simulink model "CHB2simulation2"  (R2014a)
settings: Solver=ode1  StartTime=0.0  StopTime=Tsim  FixedStep=Ts  RelTol=1e-3
InitFcn:
  | GlobalParam2;
values from neighbouring files (symbols this model uses):
  Cdc = 680e-6    (= 0.00068)    [GlobalParam2.m]
  Ideal = 1    [GlobalParam2.m]
  Rdc = 910e3    (= 910000)    [GlobalParam2.m]
  tetaa = 0    [GlobalParam2.m]
  tetab = 240    [GlobalParam2.m]
  tetac = 120    [GlobalParam2.m]
  Ts = Tm/100    (= 0.0002)    [GlobalParam2.m]
  Vdc = Vs    [GlobalParam2.m]
  Vs = 220*sqrt(2)    [GlobalParam2.m]
  we = 2*pi*fe    (= 314.159265359)    [GlobalParam2.m]
undefined symbols (not defined in the file or in its folder): Lf
libraries: powerlib x34
settings Model: Creator=Leocompa  LastModifiedBy=Leocompa

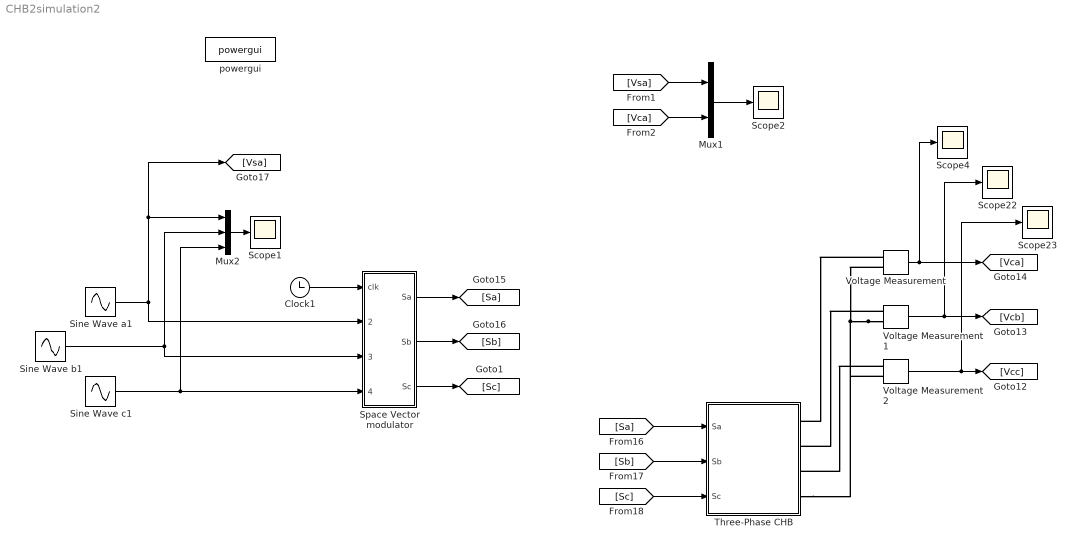
== system CHB2simulation2 ==
  Clock1 : Clock
  Mux1 : Mux  Inputs=2
  Mux2 : Mux  Inputs=3
  Scope{1..2,4,22..23} (5 alike) : Scope
      Scope1 settings: YMin=-2500  YMax=37500  SaveName=vca1
      Scope2 settings: YMin=-350  YMax=350  SaveName=vca2
      Scope22 settings: YMin=-2500  YMax=37500  SaveName=vcb
      Scope23 settings: YMin=-2500  YMax=37500  SaveName=vcc
      Scope4 settings: YMin=-2500  YMax=37500  SaveName=vca
  Sine Wave a1 : Sin  Amplitude=Vs  Frequency=we  Phase=tetaa  SampleTime=0
  Sine Wave b1 : Sin  Amplitude=Vs  Frequency=we  Phase=tetab*pi/180  SampleTime=0
  Sine Wave c1 : Sin  Amplitude=Vs  Frequency=we  Phase=tetac*pi/180  SampleTime=0
  Space Vector modulator : Subsystem
  Three-Phase CHB : Subsystem
  Voltage Measurement : powerlib/Measurements/Voltage Measurement  PhasorSimulation=off  OutputType=Complex  PSBequivalent=0
  Voltage Measurement1 : powerlib/Measurements/Voltage Measurement  PhasorSimulation=off  OutputType=Complex  PSBequivalent=0
  Voltage Measurement2 : powerlib/Measurements/Voltage Measurement  PhasorSimulation=off  OutputType=Complex  PSBequivalent=0
  powergui : powerlib/powergui  SimulationMode=Discrete  SolverType=Backward Euler  SampleTime=Ts  frequency=60  SPID=off  DisableSnubberDevices=off  DisableRonSwitches=off  DisableVfSwitches=off  SwTol=0  Interpol=off  DisplayEquations=off  Ts=0  methode=off  frequencyindice=0  Pbase=100e6  ErrMax=1e-4  Iterations=50  UnitsV=kV  UnitsW=MW  FunctionMessages=off  echomessages=off  HookPort=off  EnableUseOfTLC=off  x0status=blocks  RestoreLinks=warning  ResistiveCurrentMeasurement=off  Frange=[0:2:500]  Ylog=off  Xlog=on  ShowGrid=off  save=off  variable=ZData  structure=sa11  ZoomFFT=off  StartTime=0  cycles=8  DisplayStyle=1  fundamental=50  FreqAxis=off  MaxFrequency=10000  frequencyindicesteady=1  RmsSteady=1  display=off
  wires:
  Voltage Measurement/1 -> [Vca], Scope4/1
  Voltage Measurement2/1 -> Scope23/1, [Vcc]
  [Sa] -> Three-Phase CHB/1(Sa)
  [Sb] -> Three-Phase CHB/2(Sb)
  [Sc] -> Three-Phase CHB/3(Sc)
  Voltage Measurement1/1 -> [Vcb], Scope22/1
  [Vsa] -> Mux1/1
  [Vca] -> Mux1/2
  Mux1/1 -> Scope2/1
  Sine Wave a1/1 -> Space Vector modulator/2(vca ref), [Vsa], Mux2/1
  Sine Wave b1/1 -> Mux2/2, Space Vector modulator/3(vcb ref1)
  Sine Wave c1/1 -> Mux2/3, Space Vector modulator/4(vcc ref2)
  Mux2/1 -> Scope1/1
  Clock1/1 -> Space Vector modulator/1(clk)
  Space Vector modulator/3(Sc) -> [Sc]
  Space Vector modulator/2(Sb) -> [Sb]
  Space Vector modulator/1(Sa) -> [Sa]
  connections:
  Voltage Measurement1/LConn2 -- Voltage Measurement/LConn2 -- Three-Phase CHB/RConn4 -- Voltage Measurement2/LConn2
  Voltage Measurement2/LConn1 -- Three-Phase CHB/RConn3
  Voltage Measurement1/LConn1 -- Three-Phase CHB/RConn2
  Voltage Measurement/LConn1 -- Three-Phase CHB/RConn1

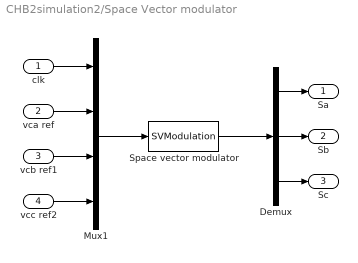
== system CHB2simulation2/Space Vector modulator ==
  clk : Inport
  vca ref : Inport  Port=2
  vcb ref1 : Inport  Port=3
  vcc ref2 : Inport  Port=4
  Demux : Demux  Outputs=3
  Mux1 : Mux
  Space vector modulator : MATLABFcn  MATLABFcn=SVModulation
  Sa : Outport
  Sb : Outport  Port=2
  Sc : Outport  Port=3
  wires:
  vcc ref2/1 -> Mux1/4
  vcb ref1/1 -> Mux1/3
  vca ref/1 -> Mux1/2
  clk/1 -> Mux1/1
  Mux1/1 -> Space vector modulator/1
  Demux/3 -> Sc/1
  Demux/2 -> Sb/1
  Demux/1 -> Sa/1
  Space vector modulator/1 -> Demux/1

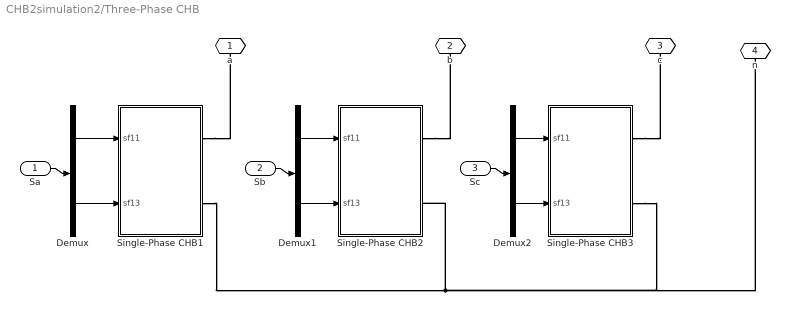
== system CHB2simulation2/Three-Phase CHB ==
  Sa : Inport
  Sb : Inport  Port=2
  Sc : Inport  Port=3
  Demux : Demux  Outputs=2
  Demux1 : Demux  Outputs=2
  Demux2 : Demux  Outputs=2
  Single-Phase CHB1 : Subsystem
  Single-Phase CHB2 : Subsystem
  Single-Phase CHB3 : Subsystem
  a : PMIOPort  Port=1  Side=Right
  b : PMIOPort  Port=2  Side=Right
  c : PMIOPort  Port=3  Side=Right
  n : PMIOPort  Port=4  Side=Right
  wires:
  Demux/2 -> Single-Phase CHB1/2(sf13)
  Demux/1 -> Single-Phase CHB1/1(sf11)
  Sa/1 -> Demux/1
  Sb/1 -> Demux1/1
  Sc/1 -> Demux2/1
  Demux2/1 -> Single-Phase CHB3/1(sf11)
  Demux1/1 -> Single-Phase CHB2/1(sf11)
  Demux1/2 -> Single-Phase CHB2/2(sf13)
  Demux2/2 -> Single-Phase CHB3/2(sf13)
  connections:
  Single-Phase CHB2/RConn1 -- b/RConn1
  Single-Phase CHB1/RConn2 -- n/RConn1 -- Single-Phase CHB3/RConn2 -- Single-Phase CHB2/RConn2
  Single-Phase CHB1/RConn1 -- a/RConn1
  Single-Phase CHB3/RConn1 -- c/RConn1

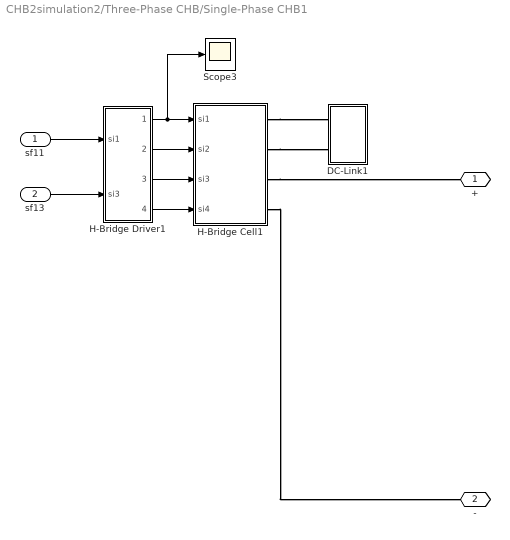
== system CHB2simulation2/Three-Phase CHB/Single-Phase CHB1 ==
  sf11 : Inport
  sf13 : Inport  Port=2
  DC-Link1 : Subsystem
  H-Bridge Cell1 : Subsystem
  H-Bridge Driver1 : Subsystem
  Scope3 : Scope
      settings: YMin=-2500  YMax=37500  SaveName=sa11
  + : PMIOPort  Port=1  Side=Right
  - : PMIOPort  Port=2  Side=Right
  wires:
  H-Bridge Driver1/1(1) -> Scope3/1, H-Bridge Cell1/1(si1)
  H-Bridge Driver1/2(2) -> H-Bridge Cell1/2(si2)
  H-Bridge Driver1/3(3) -> H-Bridge Cell1/3(si3)
  H-Bridge Driver1/4(4) -> H-Bridge Cell1/4(si4)
  sf13/1 -> H-Bridge Driver1/2(si3)
  sf11/1 -> H-Bridge Driver1/1(si1)
  connections:
  H-Bridge Cell1/RConn1 -- DC-Link1/RConn1
  H-Bridge Cell1/RConn2 -- DC-Link1/RConn2
  H-Bridge Cell1/RConn3 -- +/RConn1
  H-Bridge Cell1/RConn4 -- -/RConn1

== system CHB2simulation2/Three-Phase CHB/Single-Phase CHB2 ==
  sf11 : Inport
  sf13 : Inport  Port=2
  DC-Link1 : Subsystem
  H-Bridge Cell1 : Subsystem
  H-Bridge Driver1 : Subsystem
  + : PMIOPort  Port=1  Side=Right
  - : PMIOPort  Port=2  Side=Right
  wires:
  H-Bridge Driver1/1(1) -> H-Bridge Cell1/1(si1)
  H-Bridge Driver1/2(2) -> H-Bridge Cell1/2(si2)
  H-Bridge Driver1/3(3) -> H-Bridge Cell1/3(si3)
  H-Bridge Driver1/4(4) -> H-Bridge Cell1/4(si4)
  sf13/1 -> H-Bridge Driver1/2(si3)
  sf11/1 -> H-Bridge Driver1/1(si1)
  connections:
  DC-Link1/RConn1 -- H-Bridge Cell1/RConn1
  DC-Link1/RConn2 -- H-Bridge Cell1/RConn2
  H-Bridge Cell1/RConn3 -- +/RConn1
  H-Bridge Cell1/RConn4 -- -/RConn1

== system CHB2simulation2/Three-Phase CHB/Single-Phase CHB3 ==
  sf11 : Inport
  sf13 : Inport  Port=2
  DC-Link1 : Subsystem
  H-Bridge Cell1 : Subsystem
  H-Bridge Driver1 : Subsystem
  + : PMIOPort  Port=1  Side=Right
  - : PMIOPort  Port=2  Side=Right
  wires:
  H-Bridge Driver1/1(1) -> H-Bridge Cell1/1(si1)
  H-Bridge Driver1/2(2) -> H-Bridge Cell1/2(si2)
  H-Bridge Driver1/3(3) -> H-Bridge Cell1/3(si3)
  H-Bridge Driver1/4(4) -> H-Bridge Cell1/4(si4)
  sf13/1 -> H-Bridge Driver1/2(si3)
  sf11/1 -> H-Bridge Driver1/1(si1)
  connections:
  DC-Link1/RConn1 -- H-Bridge Cell1/RConn1
  DC-Link1/RConn2 -- H-Bridge Cell1/RConn2
  H-Bridge Cell1/RConn3 -- +/RConn1
  H-Bridge Cell1/RConn4 -- -/RConn1

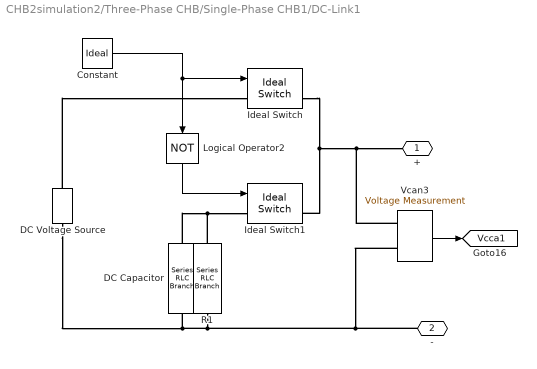
== system CHB2simulation2/Three-Phase CHB/Single-Phase CHB1/DC-Link1 ==
  Constant : Constant  Value=Ideal
  DC Capacitor : powerlib/Elements/Series RLC Branch  LConnTagsString=__new0  RConnTagsString=__new0  BranchType=C  Resistance=0.09  Inductance=0.002996  SetiL0=off  InitialCurrent=0  Capacitance=Cdc  Setx0=on  InitialVoltage=Vodc  Measurements=None
  DC Voltage Source : powerlib/Electrical Sources/DC Voltage Source  Amplitude=Vdc  Measurements=None
  Ideal Switch : powerlib/Power Electronics/Ideal Switch  Ron=0.001  Lon=0  IC=0  Rs=1e5  Cs=inf  Measurements=on
  Ideal Switch1 : powerlib/Power Electronics/Ideal Switch  Ron=0.001  Lon=0  IC=0  Rs=1e5  Cs=inf  Measurements=on
  Logical Operator2 : Logic  Operator=NOT  AllPortsSameDT=off  OutDataTypeStr=boolean
  R1 : powerlib/Elements/Series RLC Branch  LConnTagsString=__new0  RConnTagsString=__new0  BranchType=R  Resistance=Rdc  Inductance=Lf  SetiL0=off  InitialCurrent=0  Capacitance=1e-6  Setx0=off  InitialVoltage=0  Measurements=None
  Vcan3 : powerlib/Measurements/Voltage Measurement  PhasorSimulation=off  OutputType=Complex  PSBequivalent=0
  + : PMIOPort  Port=1  Side=Right
  - : PMIOPort  Port=2  Side=Right
  tag scope: Vcca1=global
  wires:
  Constant/1 -> Ideal Switch/1, Logical Operator2/1
  Logical Operator2/1 -> Ideal Switch1/1
  Vcan3/1 -> [Vcca1]
  connections:
  DC Capacitor/LConn1 -- R1/LConn1 -- Ideal Switch1/LConn1
  Ideal Switch1/RConn1 -- Ideal Switch/RConn1 -- Vcan3/LConn1 -- +/RConn1
  DC Voltage Source/RConn1 -- Ideal Switch/LConn1
  -/RConn1 -- Vcan3/LConn2 -- R1/RConn1 -- DC Voltage Source/LConn1 -- DC Capacitor/RConn1

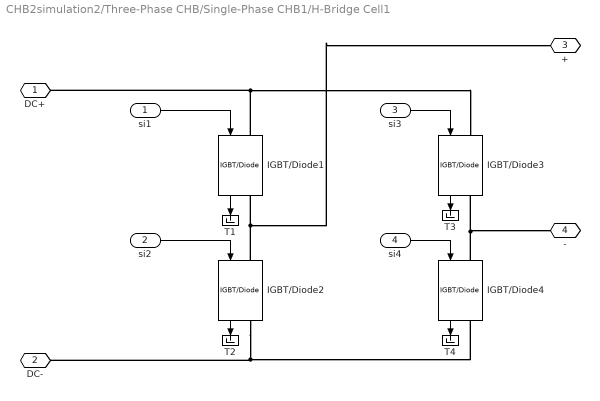
== system CHB2simulation2/Three-Phase CHB/Single-Phase CHB1/H-Bridge Cell1 ==
  si1 : Inport
  si2 : Inport  Port=2
  si3 : Inport  Port=3
  si4 : Inport  Port=4
  IGBT/Diode{1..4} (4 alike) : powerlib/Power Electronics/IGBT//Diode  Ron=1e-3  Rs=1e5  Cs=0.5  Measurements=on
  T{1..4} (4 alike) : Terminator
  DC+ : PMIOPort  Port=1  Side=Right
  DC- : PMIOPort  Port=2  Side=Right
  + : PMIOPort  Port=3  Side=Right
  - : PMIOPort  Port=4  Side=Right
  wires:
  si4/1 -> IGBT/Diode4/1
  si2/1 -> IGBT/Diode2/1
  si3/1 -> IGBT/Diode3/1
  si1/1 -> IGBT/Diode1/1
  IGBT/Diode1/1 -> T1/1
  IGBT/Diode2/1 -> T2/1
  IGBT/Diode4/1 -> T4/1
  IGBT/Diode3/1 -> T3/1
  connections:
  IGBT/Diode3/RConn1 -- IGBT/Diode4/LConn1 -- -/RConn1
  IGBT/Diode2/RConn1 -- IGBT/Diode4/RConn1 -- DC-/RConn1
  IGBT/Diode1/RConn1 -- IGBT/Diode2/LConn1 -- +/RConn1
  IGBT/Diode1/LConn1 -- IGBT/Diode3/LConn1 -- DC+/RConn1

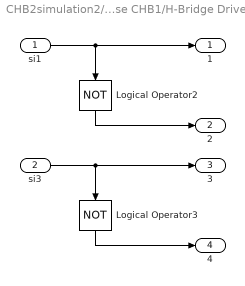
== system CHB2simulation2/Three-Phase CHB/Single-Phase CHB1/H-Bridge Driver1 ==
  si1 : Inport
  si3 : Inport  Port=2
  Logical Operator2 : Logic  Operator=NOT  AllPortsSameDT=off  OutDataTypeStr=boolean
  Logical Operator3 : Logic  Operator=NOT  AllPortsSameDT=off  OutDataTypeStr=boolean
  1 : Outport
  2 : Outport  Port=2
  3 : Outport  Port=3
  4 : Outport  Port=4
  wires:
  si3/1 -> 3/1, Logical Operator3/1
  si1/1 -> 1/1, Logical Operator2/1
  Logical Operator3/1 -> 4/1
  Logical Operator2/1 -> 2/1

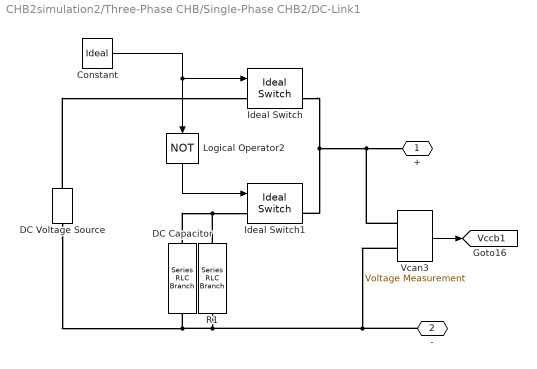
== system CHB2simulation2/Three-Phase CHB/Single-Phase CHB2/DC-Link1 ==
  Constant : Constant  Value=Ideal
  DC Capacitor : powerlib/Elements/Series RLC Branch  LConnTagsString=__new0  RConnTagsString=__new0  BranchType=C  Resistance=0.09  Inductance=0.002996  SetiL0=off  InitialCurrent=0  Capacitance=Cdc  Setx0=on  InitialVoltage=Vodc  Measurements=None
  DC Voltage Source : powerlib/Electrical Sources/DC Voltage Source  Amplitude=Vdc  Measurements=None
  Ideal Switch : powerlib/Power Electronics/Ideal Switch  Ron=0.001  Lon=0  IC=0  Rs=1e5  Cs=inf  Measurements=on
  Ideal Switch1 : powerlib/Power Electronics/Ideal Switch  Ron=0.001  Lon=0  IC=0  Rs=1e5  Cs=inf  Measurements=on
  Logical Operator2 : Logic  Operator=NOT  AllPortsSameDT=off  OutDataTypeStr=boolean
  R1 : powerlib/Elements/Series RLC Branch  LConnTagsString=__new0  RConnTagsString=__new0  BranchType=R  Resistance=Rdc  Inductance=Lf  SetiL0=off  InitialCurrent=0  Capacitance=1e-6  Setx0=off  InitialVoltage=0  Measurements=None
  Vcan3 : powerlib/Measurements/Voltage Measurement  PhasorSimulation=off  OutputType=Complex  PSBequivalent=0
  + : PMIOPort  Port=1  Side=Right
  - : PMIOPort  Port=2  Side=Right
  tag scope: Vccb1=global
  wires:
  Constant/1 -> Ideal Switch/1, Logical Operator2/1
  Logical Operator2/1 -> Ideal Switch1/1
  Vcan3/1 -> [Vccb1]
  connections:
  DC Capacitor/LConn1 -- R1/LConn1 -- Ideal Switch1/LConn1
  Ideal Switch1/RConn1 -- Ideal Switch/RConn1 -- Vcan3/LConn1 -- +/RConn1
  DC Voltage Source/RConn1 -- Ideal Switch/LConn1
  -/RConn1 -- Vcan3/LConn2 -- R1/RConn1 -- DC Capacitor/RConn1 -- DC Voltage Source/LConn1

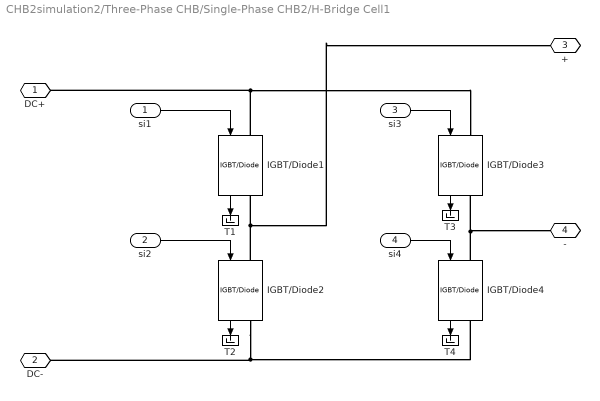
== system CHB2simulation2/Three-Phase CHB/Single-Phase CHB2/H-Bridge Cell1 ==
  si1 : Inport
  si2 : Inport  Port=2
  si3 : Inport  Port=3
  si4 : Inport  Port=4
  IGBT/Diode{1..4} (4 alike) : powerlib/Power Electronics/IGBT//Diode  Ron=1e-3  Rs=1e5  Cs=0.5  Measurements=on
  T{1..4} (4 alike) : Terminator
  DC+ : PMIOPort  Port=1  Side=Right
  DC- : PMIOPort  Port=2  Side=Right
  + : PMIOPort  Port=3  Side=Right
  - : PMIOPort  Port=4  Side=Right
  wires:
  si4/1 -> IGBT/Diode4/1
  si2/1 -> IGBT/Diode2/1
  si3/1 -> IGBT/Diode3/1
  si1/1 -> IGBT/Diode1/1
  IGBT/Diode1/1 -> T1/1
  IGBT/Diode2/1 -> T2/1
  IGBT/Diode4/1 -> T4/1
  IGBT/Diode3/1 -> T3/1
  connections:
  IGBT/Diode3/RConn1 -- IGBT/Diode4/LConn1 -- -/RConn1
  IGBT/Diode2/RConn1 -- IGBT/Diode4/RConn1 -- DC-/RConn1
  IGBT/Diode1/RConn1 -- IGBT/Diode2/LConn1 -- +/RConn1
  IGBT/Diode1/LConn1 -- IGBT/Diode3/LConn1 -- DC+/RConn1

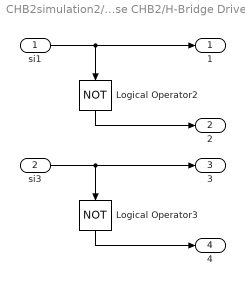
== system CHB2simulation2/Three-Phase CHB/Single-Phase CHB2/H-Bridge Driver1 ==
  si1 : Inport
  si3 : Inport  Port=2
  Logical Operator2 : Logic  Operator=NOT  AllPortsSameDT=off  OutDataTypeStr=boolean
  Logical Operator3 : Logic  Operator=NOT  AllPortsSameDT=off  OutDataTypeStr=boolean
  1 : Outport
  2 : Outport  Port=2
  3 : Outport  Port=3
  4 : Outport  Port=4
  wires:
  si3/1 -> 3/1, Logical Operator3/1
  si1/1 -> 1/1, Logical Operator2/1
  Logical Operator3/1 -> 4/1
  Logical Operator2/1 -> 2/1

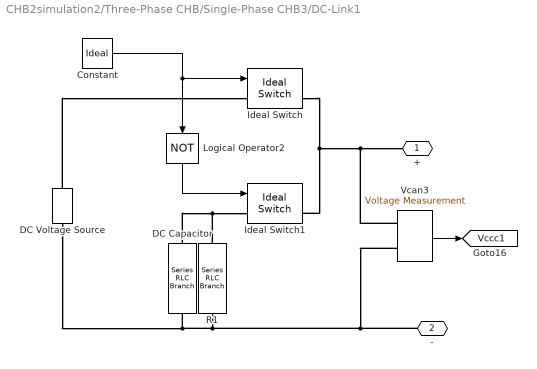
== system CHB2simulation2/Three-Phase CHB/Single-Phase CHB3/DC-Link1 ==
  Constant : Constant  Value=Ideal
  DC Capacitor : powerlib/Elements/Series RLC Branch  LConnTagsString=__new0  RConnTagsString=__new0  BranchType=C  Resistance=0.09  Inductance=0.002996  SetiL0=off  InitialCurrent=0  Capacitance=Cdc  Setx0=on  InitialVoltage=Vodc  Measurements=None
  DC Voltage Source : powerlib/Electrical Sources/DC Voltage Source  Amplitude=Vdc  Measurements=None
  Ideal Switch : powerlib/Power Electronics/Ideal Switch  Ron=0.001  Lon=0  IC=0  Rs=1e5  Cs=inf  Measurements=on
  Ideal Switch1 : powerlib/Power Electronics/Ideal Switch  Ron=0.001  Lon=0  IC=0  Rs=1e5  Cs=inf  Measurements=on
  Logical Operator2 : Logic  Operator=NOT  AllPortsSameDT=off  OutDataTypeStr=boolean
  R1 : powerlib/Elements/Series RLC Branch  LConnTagsString=__new0  RConnTagsString=__new0  BranchType=R  Resistance=Rdc  Inductance=Lf  SetiL0=off  InitialCurrent=0  Capacitance=1e-6  Setx0=off  InitialVoltage=0  Measurements=None
  Vcan3 : powerlib/Measurements/Voltage Measurement  PhasorSimulation=off  OutputType=Complex  PSBequivalent=0
  + : PMIOPort  Port=1  Side=Right
  - : PMIOPort  Port=2  Side=Right
  tag scope: Vccc1=global
  wires:
  Constant/1 -> Ideal Switch/1, Logical Operator2/1
  Logical Operator2/1 -> Ideal Switch1/1
  Vcan3/1 -> [Vccc1]
  connections:
  DC Capacitor/LConn1 -- R1/LConn1 -- Ideal Switch1/LConn1
  Ideal Switch1/RConn1 -- Ideal Switch/RConn1 -- Vcan3/LConn1 -- +/RConn1
  DC Voltage Source/RConn1 -- Ideal Switch/LConn1
  -/RConn1 -- Vcan3/LConn2 -- R1/RConn1 -- DC Capacitor/RConn1 -- DC Voltage Source/LConn1

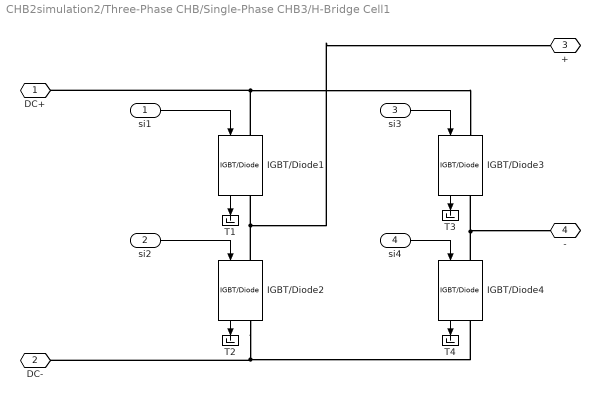
== system CHB2simulation2/Three-Phase CHB/Single-Phase CHB3/H-Bridge Cell1 ==
  si1 : Inport
  si2 : Inport  Port=2
  si3 : Inport  Port=3
  si4 : Inport  Port=4
  IGBT/Diode{1..4} (4 alike) : powerlib/Power Electronics/IGBT//Diode  Ron=1e-3  Rs=1e5  Cs=0.5  Measurements=on
  T{1..4} (4 alike) : Terminator
  DC+ : PMIOPort  Port=1  Side=Right
  DC- : PMIOPort  Port=2  Side=Right
  + : PMIOPort  Port=3  Side=Right
  - : PMIOPort  Port=4  Side=Right
  wires:
  si4/1 -> IGBT/Diode4/1
  si2/1 -> IGBT/Diode2/1
  si3/1 -> IGBT/Diode3/1
  si1/1 -> IGBT/Diode1/1
  IGBT/Diode1/1 -> T1/1
  IGBT/Diode2/1 -> T2/1
  IGBT/Diode4/1 -> T4/1
  IGBT/Diode3/1 -> T3/1
  connections:
  IGBT/Diode3/RConn1 -- IGBT/Diode4/LConn1 -- -/RConn1
  IGBT/Diode2/RConn1 -- IGBT/Diode4/RConn1 -- DC-/RConn1
  IGBT/Diode1/RConn1 -- IGBT/Diode2/LConn1 -- +/RConn1
  IGBT/Diode1/LConn1 -- IGBT/Diode3/LConn1 -- DC+/RConn1

== system CHB2simulation2/Three-Phase CHB/Single-Phase CHB3/H-Bridge Driver1 ==
  si1 : Inport
  si3 : Inport  Port=2
  Logical Operator2 : Logic  Operator=NOT  AllPortsSameDT=off  OutDataTypeStr=boolean
  Logical Operator3 : Logic  Operator=NOT  AllPortsSameDT=off  OutDataTypeStr=boolean
  1 : Outport
  2 : Outport  Port=2
  3 : Outport  Port=3
  4 : Outport  Port=4
  wires:
  si3/1 -> 3/1, Logical Operator3/1
  si1/1 -> 1/1, Logical Operator2/1
  Logical Operator3/1 -> 4/1
  Logical Operator2/1 -> 2/1
